simulink model "plant_model_fbl"  (R2023b)
settings: Solver=VariableStepAuto  StartTime=0.0  StopTime=10.0  RelTol=1e-3
undefined symbols (not defined in the file): c, d, Kp, Q_den, Q_num, R, r, sigma_n, td, Tg, Tp, Tr, tr, Tt, Tw
libraries: simulink x1
settings Model: Creator=Milosh Yokich  LastModifiedBy=Milosh Yokich

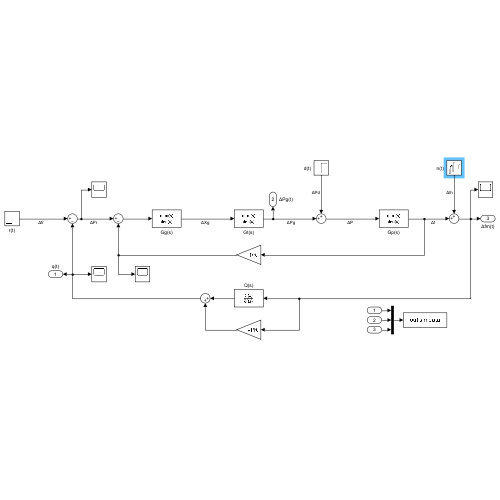
[thumbnail: Simulink's stored preview of the top-level diagram]
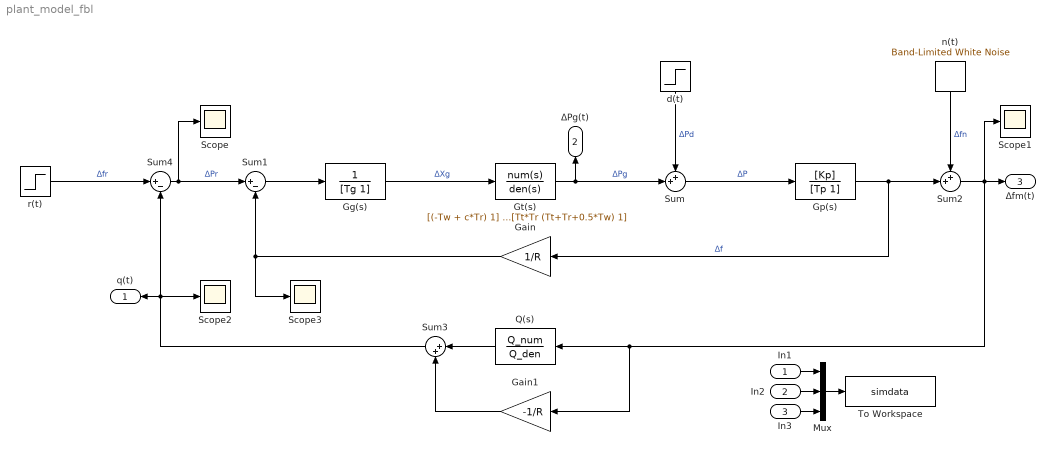
== system plant_model_fbl ==
  In1 : Inport
  In2 : Inport  Port=2
  In3 : Inport  Port=3
  Gain : Gain  Gain=1/R
  Gain1 : Gain  Gain=-1/R
  Gg(s) : TransferFcn  Denominator=[Tg 1]
  Gp(s) : TransferFcn  Numerator=[Kp]  Denominator=[Tp 1]
  Gt(s) : TransferFcn  Numerator=[(-Tw + c*Tr) 1]  Denominator=[Tt*Tr (Tt+Tr+0.5*Tw) 1]
  Mux : Mux  Inputs=3
  Q(s) : TransferFcn  Numerator=Q_num  Denominator=Q_den
  Scope{,1..3} (4 alike) : Scope
  Sum : Sum  Inputs=++|
  Sum1 : Sum  Inputs=|+-
  Sum2 : Sum  Inputs=++|
  Sum3 : Sum  Inputs=|++
  Sum4 : Sum  Inputs=|+-
  To Workspace : ToWorkspace  VariableName=simdata  SaveFormat=Timeseries  SampleTime=-1
  d(t) : Step  Time=td  After=d  SampleTime=0
  n(t) : simulink/Sources/Band-Limited White Noise  Cov=[sigma_n^2]  Ts=0.1  seed=[23341]
  r(t) : Step  Time=tr  After=r  SampleTime=0
  q(t) : Outport
  ΔPg(t) : Outport  Port=2
  Δfm(t) : Outport  Port=3
  wires:
  Gg(s)/1 -> Gt(s)/1  "ΔXg"
  Gt(s)/1 -> ΔPg(t)/1, Sum/2  "ΔPg"
  d(t)/1 -> Sum/1  "ΔPd"
  Sum/1 -> Gp(s)/1  "ΔP"
  Sum1/1 -> Gg(s)/1
  Gp(s)/1 -> Sum2/2, Gain/1  "Δf"
  Gain/1 -> Scope3/1, Sum1/2
  Sum4/1 -> Scope/1, Sum1/1  "ΔPr"
  n(t)/1 -> Sum2/1  "Δfn"
  Q(s)/1 -> Sum3/1
  Gain1/1 -> Sum3/2
  Sum2/1 -> Δfm(t)/1, Scope1/1, Gain1/1, Q(s)/1
  Sum3/1 -> Sum4/2, q(t)/1, Scope2/1
  r(t)/1 -> Sum4/1  "Δfr"
  In1/1 -> Mux/1
  In2/1 -> Mux/2
  In3/1 -> Mux/3
  Mux/1 -> To Workspace/1
